simulink library "MPSV"  (R2025b)
settings: Solver=VariableStepAuto  StartTime=0.0  StopTime=10.0  RelTol=1e-3
undefined symbols (not defined in the file or in its folder): cost, errorCode, goalReached, isFeasible, numberOfPerformedIterations, numPoses, outOfNodes, path, timestampOfComputationUTC
libraries: simulink x31, $bdroot x11, etargetslib x5
(part 3 of 3)

== system MPSV/details/Unpack Bitfield ==
  byte : Inport  OutDataTypeStr=uint8  PortDimensions=1
  Bitwise Operator : simulink/Logic and Bit Operations/Bitwise Operator  logicop=AND  UseBitMask=on  BitMask=1  BitMaskRealWorld=Stored Integer
  Bitwise Operator1 : simulink/Logic and Bit Operations/Bitwise Operator  logicop=AND  UseBitMask=on  BitMask=2  BitMaskRealWorld=Stored Integer
  Bitwise Operator2 : simulink/Logic and Bit Operations/Bitwise Operator  logicop=AND  UseBitMask=on  BitMask=4  BitMaskRealWorld=Stored Integer
  Bitwise Operator3 : simulink/Logic and Bit Operations/Bitwise Operator  logicop=AND  UseBitMask=on  BitMask=8  BitMaskRealWorld=Stored Integer
  Bitwise Operator4 : simulink/Logic and Bit Operations/Bitwise Operator  logicop=AND  UseBitMask=on  BitMask=16  BitMaskRealWorld=Stored Integer
  Bitwise Operator5 : simulink/Logic and Bit Operations/Bitwise Operator  logicop=AND  UseBitMask=on  BitMask=32  BitMaskRealWorld=Stored Integer
  Bitwise Operator6 : simulink/Logic and Bit Operations/Bitwise Operator  logicop=AND  UseBitMask=on  BitMask=64  BitMaskRealWorld=Stored Integer
  Bitwise Operator7 : simulink/Logic and Bit Operations/Bitwise Operator  logicop=AND  UseBitMask=on  BitMask=128  BitMaskRealWorld=Stored Integer
  Data Type Conversion1 : DataTypeConversion  OutDataTypeStr=boolean  SaturateOnIntegerOverflow=off  RndMeth=Floor
  Mux : Mux  Inputs=8
  bitfield : Outport  OutDataTypeStr=boolean  PortDimensions=8
  wires:
  Bitwise Operator1/1 -> Mux/2
  Bitwise Operator6/1 -> Mux/7
  Bitwise Operator7/1 -> Mux/8
  Bitwise Operator2/1 -> Mux/3
  byte/1 -> Bitwise Operator/1, Bitwise Operator7/1, Bitwise Operator6/1, Bitwise Operator5/1, Bitwise Operator4/1, Bitwise Operator3/1, Bitwise Operator2/1, Bitwise Operator1/1
  Bitwise Operator/1 -> Mux/1
  Bitwise Operator4/1 -> Mux/5
  Bitwise Operator5/1 -> Mux/6
  Bitwise Operator3/1 -> Mux/4
  Mux/1 -> Data Type Conversion1/1
  Data Type Conversion1/1 -> bitfield/1

== matlab function MPSV/Select Current Point On Trajectory/SelectPointAtTime ==
  data: success output boolean size=1; timeNow input double size=1; state output double size=9; trajectoryStartTimepoint input double size=1; sampletime input double size=1; numPoints input int32 size=1; trajectoryData input double size=[12,500]; controlInput output double size=3; remainingTrajectoryDuration output double size=1
function [success, state, controlInput, remainingTrajectoryDuration] = SelectPointAtTime(timeNow, trajectoryStartTimepoint, sampletime, numPoints, trajectoryData)
    % Set default values (invalid)
    success = false;
    state = zeros(9,1);
    controlInput = zeros(3,1);
    remainingTrajectoryDuration = 0.0;

    % Ensure correct input data
    if(~isfinite(timeNow) || ~isfinite(trajectoryStartTimepoint) || ~isfinite(sampletime) || (sampletime <= 0.0))
        return;
    end
    numPoints = int32(min(max(int32(numPoints), int32(0)), int32(size(trajectoryData,2))));

    % Calculate time difference from starting time to current time
    deltaTime = timeNow - trajectoryStartTimepoint;

    % Convert time range to sample range (including fractions of a sample)
    deltaSamples = deltaTime / sampletime;

    % Zero-order hold: get the look-up index (one-based) by rounding to the floor
    index = int32(floor(deltaSamples)) + int32(1);

    % Check the index for being in the range of the trajectory. The next point (index + 1) must also be
    % available for linear interpolation, thus the index must be in range [1, numPoints).
    if((index < int32(1)) || (index >= int32(numPoints)))
        return;
    end

    % State variables (pose, velocity, force) are set by linear interpolation
    ratio = deltaSamples - floor(deltaSamples);
    state(1) = trajectoryData(1,index) + ratio * (trajectoryData(1,(index + int32(1))) - trajectoryData(1,index));
    state(2) = trajectoryData(2,index) + ratio * (trajectoryData(2,(index + int32(1))) - trajectoryData(2,index));
    state(3) = SymmetricalAngle(trajectoryData(3,index) + ratio * SymmetricalAngle(trajectoryData(3,(index + int32(1))) - trajectoryData(3,index)));
    state(4) = trajectoryData(4,index) + ratio * (trajectoryData(4,(index + int32(1))) - trajectoryData(4,index));
    state(5) = trajectoryData(5,index) + ratio * (trajectoryData(5,(index + int32(1))) - trajectoryData(5,index));
    state(6) = trajectoryData(6,index) + ratio * (trajectoryData(6,(index + int32(1))) - trajectoryData(6,index));
    state(7) = trajectoryData(7,index) + ratio * (trajectoryData(7,(index + int32(1))) - trajectoryData(7,index));
    state(8) = trajectoryData(8,index) + ratio * (trajectoryData(8,(index + int32(1))) - trajectoryData(8,index));
    state(9) = trajectoryData(9,index) + ratio * (trajectoryData(9,(index + int32(1))) - trajectoryData(9,index));

    % Control input variables (commanded force) are set by zero-order hold
    controlInput(1) = trajectoryData(10,index);
    controlInput(2) = trajectoryData(11,index);
    controlInput(3) = trajectoryData(12,index);

    % Remaining trajectory duration from timeNow to end of trajectory (numPoints is at least 2)
    trajectoryEndTimepoint = trajectoryStartTimepoint + sampletime * double(numPoints - int32(1));
    remainingTrajectoryDuration = trajectoryEndTimepoint - timeNow;

    % Well done
    success = true;
end

function y = SymmetricalAngle(x)
    %SymmetricalAngle Convert a given angle x [rad] to an output angle y [rad] with y being in range [-pi, +pi).
    % 
    % PARAMETERS
    % x ... Input angle in radians, either scalar or n-dimensional.
    % 
    % RETURN
    % y ... Output angle in radians being in range [-pi, pi).
    x = x - 6.28318530717959 * fix(x * 0.159154943091895);
    y = x + 6.28318530717959 * double(x < -3.14159265358979) - 6.28318530717959 * double(x >= 3.14159265358979);
end

== matlab function MPSV/AutoTune AsyncOnlinePlanner/MATLAB Function ==
  data: controlEffort input double size=1; geometry_verticesVehicleShape input double size=[2,100]; geometry_collisionCheckMaxPositionDeviation input double size=1; geometry_collisionCheckMaxAngleDeviation input double size=1; model_matF input double size=[3,12]; model_matB input double size=[3,3]; model_vecSatXYN input double size=[3,1]; model_vecTimeconstantsXYN input double size=[3,1]; model_vecTimeconstantsInput input double size=[3,1]; timing_sampletime input double size=1; timing_maxComputationTimePath input double size=1; timing_maxComputationTimeMotion input double size=1; metric_weightPsi input double size=1; metric_weightSway input double size=1; metric_weightReverseScale input double size=1; metric_weightReverseDecay input double size=1; metric_distanceScale input double size=1; metric_distanceDecay input double size=1; tgeometry_skeletalPoints output double size=[2,10]; tgeometry_costMapResolution output double size=1; tgeometry_costMapModBreakpoints output int32 size=1; texplorePath_matK output double size=[3,12]; texplorePath_maxRadiusX output double size=1; texplorePath_maxRadiusY output double size=1; texplorePath_maxRadiusPsi output double size=1; texplorePath_minRadiusPosition output double size=1; texplorePath_rangePose output double size=[3,1]; texplorePath_rangeUVR output double size=[3,1]; texplorePath_rangeXYN output double size=[3,1]; tmotionPlanner_samplingRangePosition output double size=1; tmotionPlanner_samplingRangeAngle output double size=1; tmotionPlanner_maxInputPathLength output double size=1; ttiming_maxComputationTimePathOnReset output double size=1; ttiming_maxComputationTimeMotionOnReset output double size=1; ttiming_additionalAheadPlanningTime output double size=1; ttiming_additionalTrajectoryDuration output double size=1; ttiming_timeKeepPastTrajectory output double size=1; tinfo_maxUVR output double size=[3,1]; tinfo_steadyStateUVR output double size=[3,1]; errorCode output uint32 size=1
function [ ...
    tgeometry_skeletalPoints, ...
    tgeometry_costMapResolution, ...
    tgeometry_costMapModBreakpoints, ...
    texplorePath_matK, ...
    texplorePath_maxRadiusX, ...
    texplorePath_maxRadiusY, ...
    texplorePath_maxRadiusPsi, ...
    texplorePath_minRadiusPosition, ...
    texplorePath_rangePose, ...
    texplorePath_rangeUVR, ...
    texplorePath_rangeXYN, ...
    tmotionPlanner_samplingRangePosition, ...
    tmotionPlanner_samplingRangeAngle, ...
    tmotionPlanner_maxInputPathLength, ...
    ttiming_maxComputationTimePathOnReset, ...
    ttiming_maxComputationTimeMotionOnReset, ...
    ttiming_additionalAheadPlanningTime, ...
    ttiming_additionalTrajectoryDuration, ...
    ttiming_timeKeepPastTrajectory, ...
    tinfo_maxUVR, ...
    tinfo_steadyStateUVR, ...
    errorCode ...
    ] = Wrapper_MPSVDesigner( ...
    controlEffort, ...
    geometry_verticesVehicleShape, ...
    geometry_collisionCheckMaxPositionDeviation, ...
    geometry_collisionCheckMaxAngleDeviation, ...
    model_matF, ...
    model_matB, ...
    model_vecSatXYN, ...
    model_vecTimeconstantsXYN, ...
    model_vecTimeconstantsInput, ...
    timing_sampletime, ...
    timing_maxComputationTimePath, ...
    timing_maxComputationTimeMotion, ...
    metric_weightPsi, ...
    metric_weightSway, ...
    metric_weightReverseScale, ...
    metric_weightReverseDecay, ...
    metric_distanceScale, ...
    metric_distanceDecay)

    % store valid ASV settings
    persistent asv;
    if(isempty(asv))
        asv = mpsv.designer.ASV();
        asv.geometry.verticesVehicleShape = nan(2,100);
    end

    % no error code by default
    errorCode = uint32(0);

    % ensure valid controlEffort value
    if(~(IsFinite(controlEffort) && (controlEffort > 0) && (controlEffort <= 1)))
        controlEffort = 0.5;
        errorCode = errorCode + uint32(0x00000001);
    end

    % assign valid ASV settings
    if(AtLeast3FiniteVertices(geometry_verticesVehicleShape)),                     asv.geometry.verticesVehicleShape               = geometry_verticesVehicleShape;               else, errorCode = errorCode + uint32(0x00000002); end
    if(IsGreaterThanOrEqual(geometry_collisionCheckMaxPositionDeviation,0.01)),    asv.geometry.collisionCheckMaxPositionDeviation = geometry_collisionCheckMaxPositionDeviation; else, errorCode = errorCode + uint32(0x00000004); end
    if(IsGreaterThanOrEqual(geometry_collisionCheckMaxAngleDeviation,deg2rad(1))), asv.geometry.collisionCheckMaxAngleDeviation    = geometry_collisionCheckMaxAngleDeviation;    else, errorCode = errorCode + uint32(0x00000008); end
    if(IsFinite(model_matF)),                                                      asv.model.matF                                  = model_matF;                                  else, errorCode = errorCode + uint32(0x00000010); end
    if(IsFinite(model_matB)),                                                      asv.model.matB                                  = model_matB;                                  else, errorCode = errorCode + uint32(0x00000020); end
    if(IsGreaterThan(model_vecSatXYN, 0)),                                         asv.model.vecSatXYN                             = model_vecSatXYN;                             else, errorCode = errorCode + uint32(0x00000040); end
    if(IsGreaterThan(model_vecTimeconstantsXYN, 0)),                               asv.model.vecTimeconstantsXYN                   = model_vecTimeconstantsXYN;                   else, errorCode = errorCode + uint32(0x00000080); end
    if(IsGreaterThan(model_vecTimeconstantsInput, 0)),                             asv.model.vecTimeconstantsInput                 = model_vecTimeconstantsInput;                 else, errorCode = errorCode + uint32(0x00000100); end
    if(IsGreaterThan(timing_sampletime, 0)),                                       asv.timing.sampletime                           = timing_sampletime;                           else, errorCode = errorCode + uint32(0x00000200); end
    if(IsGreaterThan(timing_maxComputationTimePath, 0)),                           asv.timing.maxComputationTimePath               = timing_maxComputationTimePath;               else, errorCode = errorCode + uint32(0x00000400); end
    if(IsGreaterThan(timing_maxComputationTimePath, 0)),                           asv.timing.maxComputationTimeMotion             = timing_maxComputationTimeMotion;             else, errorCode = errorCode + uint32(0x00000800); end
    if(IsGreaterThan(metric_weightPsi, 0)),                                        asv.metric.weightPsi                            = metric_weightPsi;                            else, errorCode = errorCode + uint32(0x00001000); end
    if(IsGreaterThanOrEqual(metric_weightSway,0)),                                 asv.metric.weightSway                           = metric_weightSway;                           else, errorCode = errorCode + uint32(0x00002000); end
    if(IsGreaterThanOrEqual(metric_weightReverseScale,0)),                         asv.metric.weightReverseScale                   = metric_weightReverseScale;                   else, errorCode = errorCode + uint32(0x00004000); end
    if(IsGreaterThan(metric_weightReverseDecay, 0)),                               asv.metric.weightReverseDecay                   = metric_weightReverseDecay;                   else, errorCode = errorCode + uint32(0x00008000); end
    if(IsGreaterThanOrEqual(metric_distanceScale,0)),                              asv.metric.distanceScale                        = metric_distanceScale;                        else, errorCode = errorCode + uint32(0x00010000); end
    if(IsGreaterThan(metric_distanceDecay, 0)),                                    asv.metric.distanceDecay                        = metric_distanceDecay;                        else, errorCode = errorCode + uint32(0x00020000); end

    % do the auto tuning
    tparam = mpsv.designer.AutoTune(asv, controlEffort);

    % assign output values
    tgeometry_skeletalPoints                = tparam.geometry.skeletalPoints;
    tgeometry_costMapResolution             = tparam.geometry.costMapResolution;
    tgeometry_costMapModBreakpoints         = tparam.geometry.costMapModBreakpoints;
    texplorePath_matK                       = tparam.explorePath.matK;
    texplorePath_maxRadiusX                 = tparam.explorePath.maxRadiusX;
    texplorePath_maxRadiusY                 = tparam.explorePath.maxRadiusY;
    texplorePath_maxRadiusPsi               = tparam.explorePath.maxRadiusPsi;
    texplorePath_minRadiusPosition          = tparam.explorePath.minRadiusPosition;
    texplorePath_rangePose                  = tparam.explorePath.rangePose;
    texplorePath_rangeUVR                   = tparam.explorePath.rangeUVR;
    texplorePath_rangeXYN                   = tparam.explorePath.rangeXYN;
    tmotionPlanner_samplingRangePosition    = tparam.motionPlanner.samplingRangePosition;
    tmotionPlanner_samplingRangeAngle       = tparam.motionPlanner.samplingRangeAngle;
    tmotionPlanner_maxInputPathLength       = tparam.motionPlanner.maxInputPathLength;
    ttiming_maxComputationTimePathOnReset   = tparam.timing.maxComputationTimePathOnReset;
    ttiming_maxComputationTimeMotionOnReset = tparam.timing.maxComputationTimeMotionOnReset;
    ttiming_additionalAheadPlanningTime     = tparam.timing.additionalAheadPlanningTime;
    ttiming_additionalTrajectoryDuration    = tparam.timing.additionalTrajectoryDuration;
    ttiming_timeKeepPastTrajectory          = tparam.timing.timeKeepPastTrajectory;
    tinfo_maxUVR                            = tparam.info.maxUVR;
    tinfo_steadyStateUVR                    = tparam.info.steadyStateUVR;
end

function allValuesFinite = IsFinite(value)
    allValuesFinite = ~any(~isfinite(value),'all');
end

function allValuesPositive = IsGreaterThan(value, threshold)
    allValuesPositive = IsFinite(value) && ~any(~(value > threshold),'all');
end

function allValuesPositive = IsGreaterThanOrEqual(value, threshold)
    allValuesPositive = IsFinite(value) && ~any(~(value >= threshold),'all');
end

function finiteVertices = AtLeast3FiniteVertices(vertices)
    N = 0;
    for i = 1:size(vertices,2)
        if(isfinite(vertices(1,i)) && isfinite(vertices(2,i)))
             N = N + 1;
        end
    end
    finiteVertices = (N >= 3);
end

== matlab function MPSV/AutoTune AsyncOnlinePlanner/MATLAB Function1 ==
  data: vertices input; changed output
function changed = DetectChange(vertices)
    persistent prev_vertices;
    if(isempty(prev_vertices))
        prev_vertices = vertices;
    end
    changed = false;
    for i = 1:size(vertices,2)
        changed = ValueChanged(vertices(1,i), prev_vertices(1,i)) || ValueChanged(vertices(2,i), prev_vertices(2,i));
        if(changed)
            break;
        end
    end
    prev_vertices = vertices;
end

function a_not_b = ValueChanged(a, b)
    % Note: NaN is not equal to itself, e.g. NaN==NaN is false, NaN~=NaN is true
    a_equal_b = ((a == b) || (~isfinite(a) && ~isfinite(b)));
    a_not_b = ~a_equal_b;
end
